simulink model "test_vacc_packetise_jason"  (Simulink 6.2)
settings: Solver=ode45  StartTime=0.0  StopTime=4000  RelTol=1e-3
libraries: xbsIndex_r3 x160, xps_library x10, casper_library x8
settings Model: LastModifiedBy=dsp
settings DebuggingCC: SolverPrmCheckMsg=warning

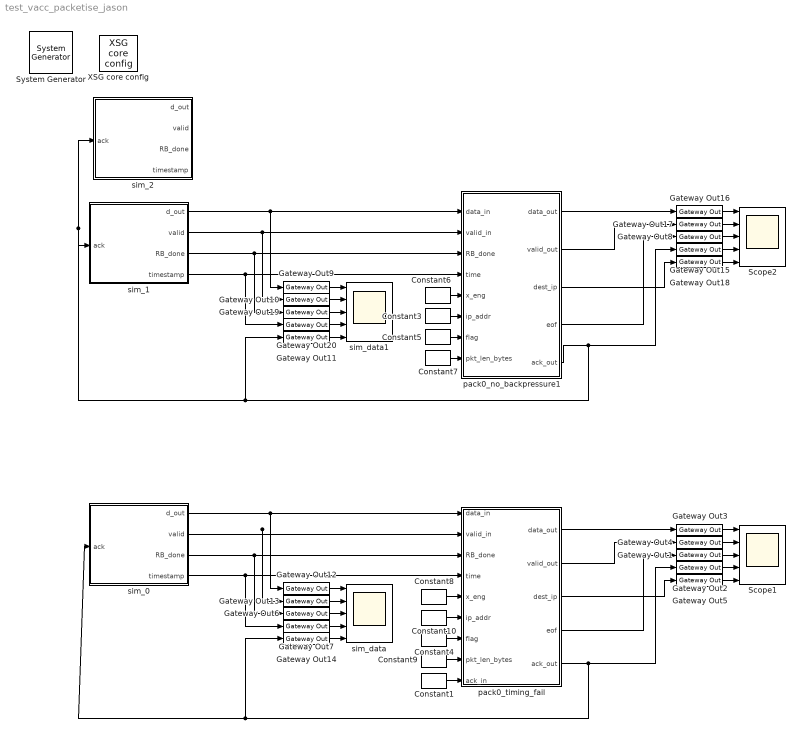
== system test_vacc_packetise_jason ==
  " System Generator" : xbsIndex_r3/ System Generator  Tag=genX  xilinxfamily=Virtex2  part=xc2v1000  speed=-4  package=bg575  synthesis_tool=XST  directory=./netlist  testbench=off  simulink_period=1  sysclk_period=100  incr_netlist=off  trim_vbits=Everywhere in SubSystem  dbl_ovrd=According to Block Masks  core_generation=According to Block Masks  run_coregen=off  deprecated_control=off  eval_field=0
      settings: AttributesFormatString=System\nGenerator
  Constant1 : xbsIndex_r3/Constant  const=1  equ=P=C  arith_type=Boolean  n_bits=32  bin_pt=0  opselect=C  inp2=PCIN>>17  opr=+  inp1=P  carry=CIN  iostate=0  explicit_period=on  period=1  dbl_ovrd=off
  Constant10 : xbsIndex_r3/Constant  const=1  equ=P=C  arith_type=Unsigned  n_bits=32  bin_pt=0  opselect=C  inp2=PCIN>>17  opr=+  inp1=P  carry=CIN  iostate=0  explicit_period=on  period=1  dbl_ovrd=off
  Constant3 : xbsIndex_r3/Constant  const=1  equ=P=C  arith_type=Unsigned  n_bits=32  bin_pt=0  opselect=C  inp2=PCIN>>17  opr=+  inp1=P  carry=CIN  iostate=0  explicit_period=on  period=1  dbl_ovrd=off
  Constant4 : xbsIndex_r3/Constant  const=0  equ=P=C  arith_type=Unsigned  n_bits=32  bin_pt=0  opselect=C  inp2=PCIN>>17  opr=+  inp1=P  carry=CIN  iostate=0  explicit_period=on  period=1  dbl_ovrd=off
  Constant5 : xbsIndex_r3/Constant  const=0  equ=P=C  arith_type=Unsigned  n_bits=32  bin_pt=0  opselect=C  inp2=PCIN>>17  opr=+  inp1=P  carry=CIN  iostate=0  explicit_period=on  period=1  dbl_ovrd=off
  Constant6 : xbsIndex_r3/Constant  const=0  equ=P=C  arith_type=Unsigned  n_bits=32  bin_pt=0  opselect=C  inp2=PCIN>>17  opr=+  inp1=P  carry=CIN  iostate=0  explicit_period=on  period=1  dbl_ovrd=off
  Constant7 : xbsIndex_r3/Constant  const=400  equ=P=C  arith_type=Unsigned  n_bits=32  bin_pt=0  opselect=C  inp2=PCIN>>17  opr=+  inp1=P  carry=CIN  iostate=0  explicit_period=on  period=1  dbl_ovrd=off
  Constant8 : xbsIndex_r3/Constant  const=0  equ=P=C  arith_type=Unsigned  n_bits=16  bin_pt=0  opselect=C  inp2=PCIN>>17  opr=+  inp1=P  carry=CIN  iostate=0  explicit_period=on  period=1  dbl_ovrd=off
  Constant9 : xbsIndex_r3/Constant  const=400  equ=P=C  arith_type=Unsigned  n_bits=32  bin_pt=0  opselect=C  inp2=PCIN>>17  opr=+  inp1=P  carry=CIN  iostate=0  explicit_period=on  period=1  dbl_ovrd=off
  Gateway Out{1..20} (20 alike) : xbsIndex_r3/Gateway Out  output_type=Double  nbits=8  bin_pt=6  arith_type=Boolean  quantization=Truncate  overflow=Wrap  hdl_port=on  timing_constraint=None  locs_specified=off  LOCs={}  needs_fixed_name=off  show_param=off
      settings: xl_area=[0, 0, 0, 0, 0, 0, 0]
  Scope1 : Scope  NumInputPorts=5
      settings: YMin=410.4~-1~-1~-1~0  YMax=453.6~1~1~1~1  SaveName=ScopeData2
  Scope2 : Scope  NumInputPorts=5
      settings: YMin=410.4~-1~-1~-1~0  YMax=453.6~1~1~1~1  SaveName=ScopeData4
  XSG core config : xps_library/XSG core config  Tag=xps:xsg  hw_sys=BEE2_usr  ibob_linux=off  clk_src=sys_clk2x  gpio_clk_io_group=iBOB:sma  gpio_clk_bit_index=0  clk_rate=205  sample_period=1  synthesis_tool=XST  mpc_type=powerpc405
  pack0_no_backpressure1 : Subsystem  mask{vector_len=100}
      mask prompts: vector_len "vector length"
  pack0_timing_fail : Subsystem  mask{vector_len=100}
      mask prompts: vector_len "vector length"
  sim_0 : Subsystem
  sim_1 : Subsystem
  sim_2 : Subsystem
  sim_data : Scope  NumInputPorts=5
      settings: YMin=0~0~0~5~0  YMax=450~1~1~7~1
  sim_data1 : Scope  NumInputPorts=5
      settings: YMin=0~0~0~5~0  YMax=450~1~1~7~1  SaveName=ScopeData5
  wires:
  Gateway Out3/1 -> Scope1/1
  Gateway Out4/1 -> Scope1/2
  Gateway Out1/1 -> Scope1/3
  Gateway Out2/1 -> Scope1/4
  Gateway Out5/1 -> Scope1/5
  sim_0/1(d_out) -> Gateway Out12/1, pack0_timing_fail/1(data_in)
  sim_0/2(valid) -> Gateway Out13/1, pack0_timing_fail/2(valid_in)
  sim_0/3(RB_done) -> Gateway Out6/1, pack0_timing_fail/3(RB_done)
  sim_0/4(timestamp) -> Gateway Out7/1, pack0_timing_fail/4(time)
  Gateway Out12/1 -> sim_data/1
  Gateway Out13/1 -> sim_data/2
  Gateway Out6/1 -> sim_data/3
  Gateway Out7/1 -> sim_data/4
  Gateway Out14/1 -> sim_data/5
  pack0_timing_fail/5(ack_out) -> Gateway Out2/1, Gateway Out14/1, sim_0/1(ack)
  Constant8/1 -> pack0_timing_fail/5(x_eng)
  Constant10/1 -> pack0_timing_fail/6(ip_addr)
  Constant4/1 -> pack0_timing_fail/7(flag)
  pack0_timing_fail/1(data_out) -> Gateway Out3/1
  pack0_timing_fail/2(valid_out) -> Gateway Out4/1
  pack0_timing_fail/4(eof) -> Gateway Out1/1
  pack0_timing_fail/3(dest_ip) -> Gateway Out5/1
  Constant9/1 -> pack0_timing_fail/8(pkt_len_bytes)
  Constant1/1 -> pack0_timing_fail/9(ack_in)
  Gateway Out16/1 -> Scope2/1
  Gateway Out17/1 -> Scope2/2
  Gateway Out8/1 -> Scope2/3
  Gateway Out15/1 -> Scope2/4
  Gateway Out18/1 -> Scope2/5
  sim_1/1(d_out) -> Gateway Out9/1, pack0_no_backpressure1/1(data_in)
  sim_1/2(valid) -> Gateway Out10/1, pack0_no_backpressure1/2(valid_in)
  sim_1/3(RB_done) -> Gateway Out19/1, pack0_no_backpressure1/3(RB_done)
  sim_1/4(timestamp) -> Gateway Out20/1, pack0_no_backpressure1/4(time)
  Gateway Out9/1 -> sim_data1/1
  Gateway Out10/1 -> sim_data1/2
  Gateway Out19/1 -> sim_data1/3
  Gateway Out20/1 -> sim_data1/4
  Gateway Out11/1 -> sim_data1/5
  pack0_no_backpressure1/5(ack_out) -> Gateway Out11/1, sim_1/1(ack), sim_2/1(ack), Gateway Out15/1
  pack0_no_backpressure1/1(data_out) -> Gateway Out16/1
  pack0_no_backpressure1/2(valid_out) -> Gateway Out17/1
  pack0_no_backpressure1/4(eof) -> Gateway Out8/1
  pack0_no_backpressure1/3(dest_ip) -> Gateway Out18/1
  Constant6/1 -> pack0_no_backpressure1/5(x_eng)
  Constant3/1 -> pack0_no_backpressure1/6(ip_addr)
  Constant5/1 -> pack0_no_backpressure1/7(flag)
  Constant7/1 -> pack0_no_backpressure1/8(pkt_len_bytes)

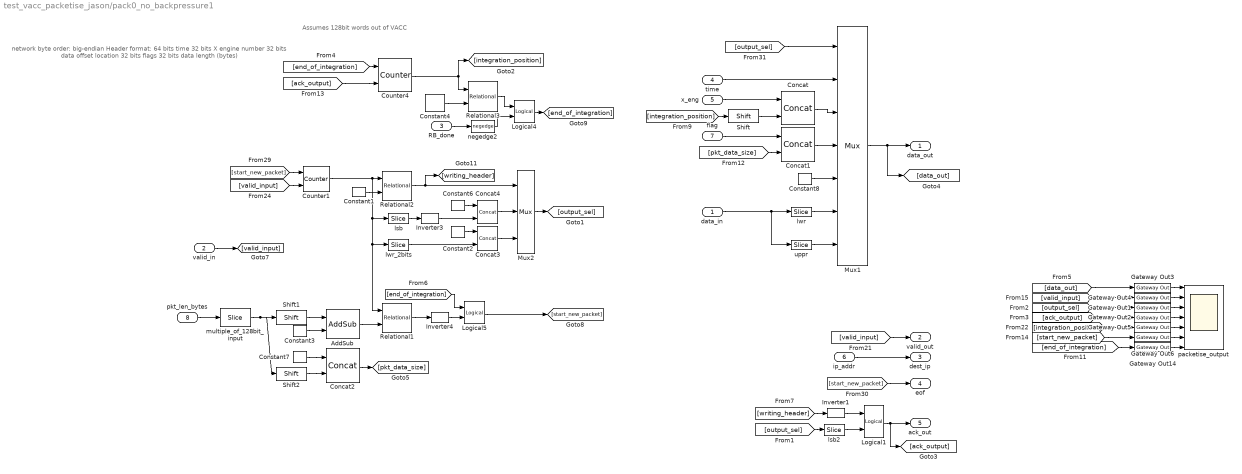
== system test_vacc_packetise_jason/pack0_no_backpressure1 ==
  note: network byte order: big-endian
      |
      | Header format:
      | 64 bits time
      | 32 bits X engine number
      | 32 bits data offset location
      | 32 bits flags
      | 32 bits data length (bytes)
  note: Assumes 128bit words out of VACC
  data_in : Inport  Port=1  LatchInput=off
  valid_in : Inport  Port=2  LatchInput=off
  RB_done : Inport  Port=3  LatchInput=off
  time : Inport  Port=4  LatchInput=off
  x_eng : Inport  Port=5  LatchInput=off
  ip_addr : Inport  Port=6  LatchInput=off
  flag : Inport  Port=7  LatchInput=off
  pkt_len_bytes : Inport  Port=8  LatchInput=off
  AddSub : xbsIndex_r3/AddSub  mode=Addition  precision=Full  arith_type=Unsigned  n_bits=8  bin_pt=2  quantization=Truncate  overflow=Wrap  latency=2  explicit_period=on  period=1  use_carryin=off  use_carryout=off  en=off  dbl_ovrd=off  show_param=off  use_core=on  pipeline=off  use_rpm=on  gen_core=off
      settings: xl_area=[0, 0, 0, 0, 0, 0, 0]
  Concat : xbsIndex_r3/Concat  num_inputs=2  explicit_period=on  period=1  dbl_ovrd=off
  Concat{1..4} (4 alike) : xbsIndex_r3/Concat  num_inputs=2  explicit_period=off  period=1  dbl_ovrd=off
  Constant1 : xbsIndex_r3/Constant  const=2  equ=P=C  arith_type=Unsigned  n_bits=2  bin_pt=0  opselect=C  inp2=PCIN>>17  opr=+  inp1=P  carry=CIN  iostate=0  explicit_period=on  period=1  dbl_ovrd=off
  Constant2 : xbsIndex_r3/Constant  const=0  equ=P=C  arith_type=Unsigned  n_bits=1  bin_pt=0  opselect=C  inp2=PCIN>>17  opr=+  inp1=P  carry=CIN  iostate=0  explicit_period=on  period=1  dbl_ovrd=off
  Constant3 : xbsIndex_r3/Constant  const=2  equ=P=C  arith_type=Unsigned  n_bits=32  bin_pt=0  opselect=C  inp2=PCIN>>17  opr=+  inp1=P  carry=CIN  iostate=0  explicit_period=on  period=1  dbl_ovrd=off
  Constant4 : xbsIndex_r3/Constant  const=2*vector_len-1  equ=P=C  arith_type=Unsigned  n_bits=32  bin_pt=0  opselect=C  inp2=PCIN>>17  opr=+  inp1=P  carry=CIN  iostate=0  explicit_period=off  period=1  dbl_ovrd=off
  Constant6 : xbsIndex_r3/Constant  const=2  equ=P=C  arith_type=Unsigned  n_bits=2  bin_pt=0  opselect=C  inp2=PCIN>>17  opr=+  inp1=P  carry=CIN  iostate=0  explicit_period=on  period=1  dbl_ovrd=off
  Constant7 : xbsIndex_r3/Constant  const=0  equ=P=C  arith_type=Unsigned  n_bits=32-28  bin_pt=0  opselect=C  inp2=PCIN>>17  opr=+  inp1=P  carry=CIN  iostate=0  explicit_period=on  period=1  dbl_ovrd=off
  Constant8 : xbsIndex_r3/Constant  const=0  equ=P=C  arith_type=Unsigned  n_bits=64  bin_pt=0  opselect=C  inp2=PCIN>>17  opr=+  inp1=P  carry=CIN  iostate=0  explicit_period=on  period=1  dbl_ovrd=off
  Counter1 : xbsIndex_r3/Counter  cnt_type=Free Running  n_bits=32  bin_pt=0  arith_type=Unsigned  start_count=0  cnt_to=1023  cnt_by_val=1  operation=Up  explicit_period=on  period=1  load_pin=off  rst=on  en=on  dbl_ovrd=off  show_param=off  use_rpm=on  gen_core=off
      settings: xl_area=[0, 0, 0, 0, 0, 0, 0]
  Counter4 : xbsIndex_r3/Counter  cnt_type=Free Running  n_bits=32  bin_pt=0  arith_type=Unsigned  start_count=0  cnt_to=1023  cnt_by_val=1  operation=Up  explicit_period=on  period=1  load_pin=off  rst=on  en=on  dbl_ovrd=off  show_param=off  use_rpm=on  gen_core=off
      settings: xl_area=[0, 0, 0, 0, 0, 0, 0]
  Gateway Out{1..6,14} (7 alike) : xbsIndex_r3/Gateway Out  output_type=Double  nbits=8  bin_pt=6  arith_type=Boolean  quantization=Truncate  overflow=Wrap  hdl_port=on  timing_constraint=None  locs_specified=off  LOCs={}  needs_fixed_name=off  show_param=off
      settings: xl_area=[0, 0, 0, 0, 0, 0, 0]
  Inverter1 : xbsIndex_r3/Inverter  latency=0  explicit_period=off  period=1  en=off  dbl_ovrd=off  show_param=off
      settings: xl_area=[0, 0, 0, 0, 0, 0, 0]
  Inverter3 : xbsIndex_r3/Inverter  latency=0  explicit_period=off  period=1  en=off  dbl_ovrd=off  show_param=off
      settings: xl_area=[0, 0, 0, 0, 0, 0, 0]
  Inverter4 : xbsIndex_r3/Inverter  latency=0  explicit_period=off  period=1  en=off  dbl_ovrd=off  show_param=off
      settings: xl_area=[0, 0, 0, 0, 0, 0, 0]
  Logical1 : xbsIndex_r3/Logical  logical_function=AND  inputs=2  precision=Full  arith_type=Unsigned  n_bits=8  bin_pt=2  align_bp=on  latency=0  explicit_period=off  period=1  en=off  dbl_ovrd=off  show_param=off
      settings: xl_area=[0, 0, 0, 0, 0, 0, 0]
  Logical4 : xbsIndex_r3/Logical  logical_function=OR  inputs=2  precision=Full  arith_type=Unsigned  n_bits=8  bin_pt=2  align_bp=on  latency=0  explicit_period=off  period=1  en=off  dbl_ovrd=off  show_param=off
      settings: xl_area=[0, 0, 0, 0, 0, 0, 0]
  Logical5 : xbsIndex_r3/Logical  logical_function=OR  inputs=2  precision=Full  arith_type=Unsigned  n_bits=8  bin_pt=2  align_bp=on  latency=0  explicit_period=off  period=1  en=off  dbl_ovrd=off  show_param=off
      settings: xl_area=[0, 0, 0, 0, 0, 0, 0]
  Mux1 : xbsIndex_r3/Mux  inputs=6  precision=Full  arith_type="Signed  (2's comp)"  n_bits=8  bin_pt=2  quantization=Truncate  overflow=Wrap  latency=0  explicit_period=off  period=1  en=off  dbl_ovrd=off  show_param=off  mux_type=off  use_rpm=off  gen_core=off
      settings: xl_area=[0, 0, 0, 0, 0, 0, 0]
  Mux2 : xbsIndex_r3/Mux  inputs=2  precision=Full  arith_type="Signed  (2's comp)"  n_bits=8  bin_pt=2  quantization=Truncate  overflow=Wrap  latency=0  explicit_period=off  period=1  en=off  dbl_ovrd=off  show_param=off  mux_type=off  use_rpm=off  gen_core=off
      settings: xl_area=[0, 0, 0, 0, 0, 0, 0]
  Relational1 : xbsIndex_r3/Relational  mode=a<=b  latency=0  explicit_period=off  period=1  en=off  dbl_ovrd=off  show_param=off
      settings: xl_area=[0, 0, 0, 0, 0, 0, 0]
  Relational2 : xbsIndex_r3/Relational  mode=a<=b  latency=0  explicit_period=off  period=1  en=off  dbl_ovrd=off  show_param=off
      settings: xl_area=[0, 0, 0, 0, 0, 0, 0]
  Relational3 : xbsIndex_r3/Relational  mode=a>=b  latency=0  explicit_period=off  period=1  en=off  dbl_ovrd=off  show_param=off
      settings: xl_area=[0, 0, 0, 0, 0, 0, 0]
  Shift : xbsIndex_r3/Shift  shift_dir=Left  shift_bits=4  precision=Full  arith_type="Signed  (2's comp)"  n_bits=8  bin_pt=2  quantization=Truncate  overflow=Wrap  latency=0  explicit_period=off  period=1  en=off  dbl_ovrd=off  show_param=off
      settings: xl_area=[0, 0, 0, 0, 0, 0, 0]
  Shift1 : xbsIndex_r3/Shift  shift_dir=Left  shift_bits=1  precision=Full  arith_type="Signed  (2's comp)"  n_bits=8  bin_pt=2  quantization=Truncate  overflow=Wrap  latency=2  explicit_period=on  period=1  en=off  dbl_ovrd=off  show_param=off
      settings: xl_area=[0, 0, 0, 0, 0, 0, 0]
  Shift2 : xbsIndex_r3/Shift  shift_dir=Left  shift_bits=4  precision=Full  arith_type="Signed  (2's comp)"  n_bits=8  bin_pt=2  quantization=Truncate  overflow=Wrap  latency=2  explicit_period=on  period=1  en=off  dbl_ovrd=off  show_param=off
      settings: xl_area=[0, 0, 0, 0, 0, 0, 0]
  lsb : xbsIndex_r3/Slice  mode=Lower Bit Location + Width  nbits=1  bit1=0  base1=MSB of Input  bit0=0  base0=LSB of Input  boolean_output=off  explicit_period=off  period=1  dbl_ovrd=off
  lsb2 : xbsIndex_r3/Slice  mode=Lower Bit Location + Width  nbits=1  bit1=0  base1=MSB of Input  bit0=0  base0=LSB of Input  boolean_output=on  explicit_period=off  period=1  dbl_ovrd=off
  lwr : xbsIndex_r3/Slice  mode=Lower Bit Location + Width  nbits=64  bit1=0  base1=MSB of Input  bit0=0  base0=LSB of Input  boolean_output=off  explicit_period=off  period=1  dbl_ovrd=off
  lwr_2bits : xbsIndex_r3/Slice  mode=Lower Bit Location + Width  nbits=2  bit1=0  base1=MSB of Input  bit0=0  base0=LSB of Input  boolean_output=on  explicit_period=off  period=1  dbl_ovrd=off
  multiple_of_128bit_input : xbsIndex_r3/Slice  mode=Two Bit Locations  nbits=64  bit1=31  base1=LSB of Input  bit0=4  base0=LSB of Input  boolean_output=off  explicit_period=off  period=1  dbl_ovrd=off
  negedge2 : casper_library/Misc/negedge  Tag=Rising Edge Detector
  packetise_output : Scope  NumInputPorts=7
      settings: YMin=0~0~0~0~0~0~0  YMax=1200~1~5~1~100~1~1
  uppr : xbsIndex_r3/Slice  mode=Upper Bit Location + Width  nbits=64  bit1=0  base1=MSB of Input  bit0=0  base0=LSB of Input  boolean_output=off  explicit_period=off  period=1  dbl_ovrd=off
  data_out : Outport
  valid_out : Outport  Port=2
  dest_ip : Outport  Port=3
  eof : Outport  Port=4
  ack_out : Outport  Port=5
  wires:
  [ack_output] -> Gateway Out2/1
  AddSub/1 -> Relational1/2
  Shift1/1 -> AddSub/1
  multiple_of_128bit_input/1 -> Shift2/1, Shift1/1
  pkt_len_bytes/1 -> multiple_of_128bit_input/1
  Inverter4/1 -> Logical5/2
  [integration_position] -> Gateway Out5/1
  [end_of_integration] -> Gateway Out14/1
  Gateway Out14/1 -> packetise_output/7
  [valid_input] -> valid_out/1
  [valid_input] -> Gateway Out4/1
  [start_new_packet] -> Gateway Out6/1
  [end_of_integration] -> Logical5/1
  Relational1/1 -> Inverter4/1
  Gateway Out6/1 -> packetise_output/6
  Gateway Out5/1 -> packetise_output/5
  Gateway Out2/1 -> packetise_output/4
  Gateway Out1/1 -> packetise_output/3
  Gateway Out4/1 -> packetise_output/2
  Gateway Out3/1 -> packetise_output/1
  ip_addr/1 -> dest_ip/1
  valid_in/1 -> [valid_input]
  Mux1/1 -> data_out/1, [data_out]
  Logical5/1 -> [start_new_packet]
  Counter1/1 -> Relational2/1, lwr_2bits/1, Relational1/1, lsb/1
  [valid_input] -> Counter1/2
  Constant3/1 -> AddSub/2
  [start_new_packet] -> Counter1/1
  [start_new_packet] -> eof/1
  Relational2/1 -> [writing_header], Mux2/1
  Constant1/1 -> Relational2/2
  Mux2/1 -> [output_sel]
  [output_sel] -> lsb2/1
  Concat2/1 -> [pkt_data_size]
  Shift2/1 -> Concat2/2
  Constant7/1 -> Concat2/1
  [output_sel] -> Mux1/1
  Concat3/1 -> Mux2/3
  lwr_2bits/1 -> Concat3/2
  Constant2/1 -> Concat3/1
  lsb/1 -> Inverter3/1
  Constant6/1 -> Concat4/1
  Concat4/1 -> Mux2/2
  [end_of_integration] -> Counter4/1
  Counter4/1 -> [integration_position], Relational3/1
  [ack_output] -> Counter4/2
  [output_sel] -> Gateway Out1/1
  [data_out] -> Gateway Out3/1
  Logical1/1 -> ack_out/1, [ack_output]
  lsb2/1 -> Logical1/2
  Inverter1/1 -> Logical1/1
  [writing_header] -> Inverter1/1
  Inverter3/1 -> Concat4/2
  Constant4/1 -> Relational3/2
  Logical4/1 -> [end_of_integration]
  Relational3/1 -> Logical4/1
  negedge2/1 -> Logical4/2
  RB_done/1 -> negedge2/1
  data_in/1 -> lwr/1, uppr/1
  lwr/1 -> Mux1/6
  uppr/1 -> Mux1/7
  Constant8/1 -> Mux1/5
  Shift/1 -> Concat/2
  [pkt_data_size] -> Concat1/2
  flag/1 -> Concat1/1
  [integration_position] -> Shift/1
  x_eng/1 -> Concat/1
  Concat1/1 -> Mux1/4
  Concat/1 -> Mux1/3
  time/1 -> Mux1/2

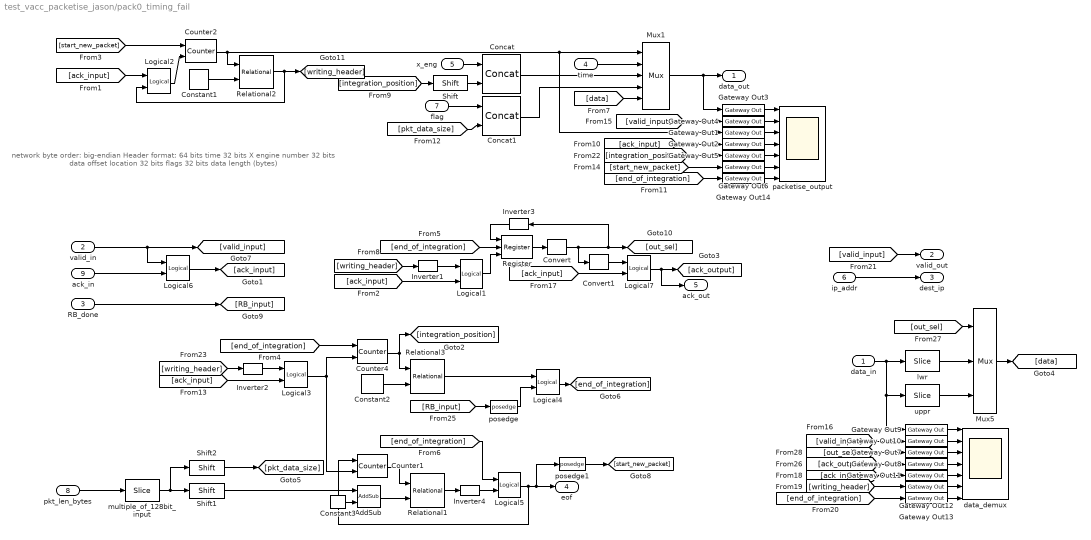
== system test_vacc_packetise_jason/pack0_timing_fail ==
  note: network byte order: big-endian
      |
      | Header format:
      | 64 bits time
      | 32 bits X engine number
      | 32 bits data offset location
      | 32 bits flags
      | 32 bits data length (bytes)
  data_in : Inport  Port=1  LatchInput=off
  valid_in : Inport  Port=2  LatchInput=off
  RB_done : Inport  Port=3  LatchInput=off
  time : Inport  Port=4  LatchInput=off
  x_eng : Inport  Port=5  LatchInput=off
  ip_addr : Inport  Port=6  LatchInput=off
  flag : Inport  Port=7  LatchInput=off
  pkt_len_bytes : Inport  Port=8  LatchInput=off
  ack_in : Inport  Port=9  LatchInput=off
  AddSub : xbsIndex_r3/AddSub  mode=Subtraction  precision=Full  arith_type=Unsigned  n_bits=8  bin_pt=2  quantization=Truncate  overflow=Wrap  latency=2  explicit_period=on  period=1  use_carryin=off  use_carryout=off  en=off  dbl_ovrd=off  show_param=off  use_core=on  pipeline=off  use_rpm=on  gen_core=off
      settings: xl_area=[0, 0, 0, 0, 0, 0, 0]
  Concat : xbsIndex_r3/Concat  num_inputs=2  explicit_period=off  period=1  dbl_ovrd=off
  Concat1 : xbsIndex_r3/Concat  num_inputs=2  explicit_period=off  period=1  dbl_ovrd=off
  Constant1 : xbsIndex_r3/Constant  const=2  equ=P=C  arith_type=Unsigned  n_bits=2  bin_pt=0  opselect=C  inp2=PCIN>>17  opr=+  inp1=P  carry=CIN  iostate=0  explicit_period=off  period=1  dbl_ovrd=off
  Constant2 : xbsIndex_r3/Constant  const=2*vector_len-1  equ=P=C  arith_type=Unsigned  n_bits=32  bin_pt=0  opselect=C  inp2=PCIN>>17  opr=+  inp1=P  carry=CIN  iostate=0  explicit_period=off  period=1  dbl_ovrd=off
  Constant3 : xbsIndex_r3/Constant  const=2  equ=P=C  arith_type=Unsigned  n_bits=32  bin_pt=0  opselect=C  inp2=PCIN>>17  opr=+  inp1=P  carry=CIN  iostate=0  explicit_period=off  period=1  dbl_ovrd=off
  Convert : xbsIndex_r3/Convert  arith_type=Unsigned  n_bits=1  bin_pt=0  quantization=Truncate  overflow=Wrap  latency=0  explicit_period=off  period=1  dbl_ovrd=off  show_param=off  inserted_by_tool=off  pipeline=off
      settings: xl_area=[0, 0, 0, 0, 0, 0, 0]
  Convert1 : xbsIndex_r3/Convert  arith_type=Boolean  n_bits=1  bin_pt=0  quantization=Truncate  overflow=Wrap  latency=0  explicit_period=off  period=1  dbl_ovrd=off  show_param=off  inserted_by_tool=off  pipeline=off
      settings: xl_area=[0, 0, 0, 0, 0, 0, 0]
  Counter1 : xbsIndex_r3/Counter  cnt_type=Free Running  n_bits=32  bin_pt=0  arith_type=Unsigned  start_count=0  cnt_to=1023  cnt_by_val=1  operation=Up  explicit_period=on  period=1  load_pin=off  rst=on  en=on  dbl_ovrd=off  show_param=off  use_rpm=on  gen_core=off
      settings: xl_area=[0, 0, 0, 0, 0, 0, 0]
  Counter2 : xbsIndex_r3/Counter  cnt_type=Free Running  n_bits=2  bin_pt=0  arith_type=Unsigned  start_count=0  cnt_to=1023  cnt_by_val=1  operation=Up  explicit_period=on  period=1  load_pin=off  rst=on  en=on  dbl_ovrd=off  show_param=off  use_rpm=on  gen_core=off
      settings: xl_area=[0, 0, 0, 0, 0, 0, 0]
  Counter4 : xbsIndex_r3/Counter  cnt_type=Free Running  n_bits=32  bin_pt=0  arith_type=Unsigned  start_count=0  cnt_to=1023  cnt_by_val=1  operation=Up  explicit_period=on  period=1  load_pin=off  rst=on  en=on  dbl_ovrd=off  show_param=off  use_rpm=on  gen_core=off
      settings: xl_area=[0, 0, 0, 0, 0, 0, 0]
  Gateway Out{1..14} (14 alike) : xbsIndex_r3/Gateway Out  output_type=Double  nbits=8  bin_pt=6  arith_type=Boolean  quantization=Truncate  overflow=Wrap  hdl_port=on  timing_constraint=None  locs_specified=off  LOCs={}  needs_fixed_name=off  show_param=off
      settings: xl_area=[0, 0, 0, 0, 0, 0, 0]
  Inverter1 : xbsIndex_r3/Inverter  latency=0  explicit_period=off  period=1  en=off  dbl_ovrd=off  show_param=off
      settings: xl_area=[0, 0, 0, 0, 0, 0, 0]
  Inverter2 : xbsIndex_r3/Inverter  latency=0  explicit_period=off  period=1  en=off  dbl_ovrd=off  show_param=off
      settings: xl_area=[0, 0, 0, 0, 0, 0, 0]
  Inverter3 : xbsIndex_r3/Inverter  Orientation=left  latency=0  explicit_period=on  period=1  en=off  dbl_ovrd=off  show_param=off
      settings: xl_area=[0, 0, 0, 0, 0, 0, 0]
  Inverter4 : xbsIndex_r3/Inverter  latency=0  explicit_period=off  period=1  en=off  dbl_ovrd=off  show_param=off
      settings: xl_area=[0, 0, 0, 0, 0, 0, 0]
  Logical{1..3,6..7} (5 alike) : xbsIndex_r3/Logical  logical_function=AND  inputs=2  precision=Full  arith_type=Unsigned  n_bits=8  bin_pt=2  align_bp=on  latency=0  explicit_period=off  period=1  en=off  dbl_ovrd=off  show_param=off
      settings: xl_area=[0, 0, 0, 0, 0, 0, 0]
  Logical4 : xbsIndex_r3/Logical  logical_function=OR  inputs=2  precision=Full  arith_type=Unsigned  n_bits=8  bin_pt=2  align_bp=on  latency=0  explicit_period=off  period=1  en=off  dbl_ovrd=off  show_param=off
      settings: xl_area=[0, 0, 0, 0, 0, 0, 0]
  Logical5 : xbsIndex_r3/Logical  logical_function=OR  inputs=2  precision=Full  arith_type=Unsigned  n_bits=8  bin_pt=2  align_bp=on  latency=0  explicit_period=off  period=1  en=off  dbl_ovrd=off  show_param=off
      settings: xl_area=[0, 0, 0, 0, 0, 0, 0]
  Mux1 : xbsIndex_r3/Mux  inputs=4  precision=Full  arith_type="Signed  (2's comp)"  n_bits=8  bin_pt=2  quantization=Truncate  overflow=Wrap  latency=0  explicit_period=off  period=1  en=off  dbl_ovrd=off  show_param=off  mux_type=off  use_rpm=off  gen_core=off
      settings: xl_area=[0, 0, 0, 0, 0, 0, 0]
  Mux5 : xbsIndex_r3/Mux  inputs=2  precision=Full  arith_type="Signed  (2's comp)"  n_bits=8  bin_pt=2  quantization=Truncate  overflow=Wrap  latency=0  explicit_period=on  period=1  en=off  dbl_ovrd=off  show_param=off  mux_type=off  use_rpm=off  gen_core=off
      settings: xl_area=[0, 0, 0, 0, 0, 0, 0]
  Register : xbsIndex_r3/Register  init=0  reg_only_valid=off  explicit_period=on  period=1  rst=on  en=on  out_en=off  dbl_ovrd=off  show_param=off
      settings: xl_area=[0, 0, 0, 0, 0, 0, 0]
  Relational1 : xbsIndex_r3/Relational  mode=a<=b  latency=0  explicit_period=off  period=1  en=off  dbl_ovrd=off  show_param=off
      settings: xl_area=[0, 0, 0, 0, 0, 0, 0]
  Relational2 : xbsIndex_r3/Relational  mode=a<=b  latency=0  explicit_period=off  period=1  en=off  dbl_ovrd=off  show_param=off
      settings: xl_area=[0, 0, 0, 0, 0, 0, 0]
  Relational3 : xbsIndex_r3/Relational  mode=a>=b  latency=0  explicit_period=off  period=1  en=off  dbl_ovrd=off  show_param=off
      settings: xl_area=[0, 0, 0, 0, 0, 0, 0]
  Shift : xbsIndex_r3/Shift  shift_dir=Left  shift_bits=3  precision=Full  arith_type="Signed  (2's comp)"  n_bits=8  bin_pt=2  quantization=Truncate  overflow=Wrap  latency=0  explicit_period=off  period=1  en=off  dbl_ovrd=off  show_param=off
      settings: xl_area=[0, 0, 0, 0, 0, 0, 0]
  Shift1 : xbsIndex_r3/Shift  shift_dir=Left  shift_bits=1  precision=Full  arith_type="Signed  (2's comp)"  n_bits=8  bin_pt=2  quantization=Truncate  overflow=Wrap  latency=2  explicit_period=on  period=1  en=off  dbl_ovrd=off  show_param=off
      settings: xl_area=[0, 0, 0, 0, 0, 0, 0]
  Shift2 : xbsIndex_r3/Shift  shift_dir=Left  shift_bits=4  precision=Full  arith_type="Signed  (2's comp)"  n_bits=8  bin_pt=2  quantization=Truncate  overflow=Wrap  latency=2  explicit_period=on  period=1  en=off  dbl_ovrd=off  show_param=off
      settings: xl_area=[0, 0, 0, 0, 0, 0, 0]
  data_demux : Scope  NumInputPorts=7
      settings: YMin=410.4~-1~-1~-1~0~-5~-5  YMax=453.6~1~1~1~1~5~5  SaveName=ScopeData3
  lwr : xbsIndex_r3/Slice  mode=Lower Bit Location + Width  nbits=64  bit1=0  base1=MSB of Input  bit0=0  base0=LSB of Input  boolean_output=off  explicit_period=off  period=1  dbl_ovrd=off
  multiple_of_128bit_input : xbsIndex_r3/Slice  mode=Two Bit Locations  nbits=64  bit1=0  base1=MSB of Input  bit0=4  base0=LSB of Input  boolean_output=off  explicit_period=off  period=1  dbl_ovrd=off
  packetise_output : Scope  NumInputPorts=7
      settings: YMin=410.4~-1~-1~-1~0~-5~-5  YMax=453.6~1~1~1~1~5~5
  posedge : casper_library/Misc/posedge  Tag=Rising Edge Detector
  posedge1 : casper_library/Misc/posedge  Tag=Rising Edge Detector
  uppr : xbsIndex_r3/Slice  mode=Upper Bit Location + Width  nbits=64  bit1=0  base1=MSB of Input  bit0=0  base0=LSB of Input  boolean_output=off  explicit_period=off  period=1  dbl_ovrd=off
  data_out : Outport
  valid_out : Outport  Port=2
  dest_ip : Outport  Port=3
  eof : Outport  Port=4
  ack_out : Outport  Port=5
  wires:
  lwr/1 -> Mux5/2
  uppr/1 -> Mux5/3
  [ack_input] -> Logical1/2
  Counter1/1 -> Relational1/1
  Logical5/1 -> Counter1/1, eof/1, posedge1/1
  Constant1/1 -> Relational2/2
  Counter2/1 -> Relational2/1, Mux1/1, Gateway Out1/1
  time/1 -> Mux1/2
  Logical2/1 -> Counter2/2
  Relational2/1 -> Logical2/2, [writing_header]
  [ack_input] -> Logical2/1
  [start_new_packet] -> Counter2/1
  [end_of_integration] -> Counter4/1
  Counter4/1 -> [integration_position], Relational3/1
  Mux1/1 -> data_out/1, Gateway Out3/1
  Mux5/1 -> [data]
  [writing_header] -> Inverter1/1
  Inverter1/1 -> Logical1/1
  x_eng/1 -> Concat/1
  [integration_position] -> Shift/1
  Concat/1 -> Mux1/3
  valid_in/1 -> [valid_input], Logical6/1
  ip_addr/1 -> dest_ip/1
  flag/1 -> Concat1/1
  [pkt_data_size] -> Concat1/2
  Concat1/1 -> Mux1/4
  Logical3/1 -> Counter4/2, Counter1/2
  Gateway Out3/1 -> packetise_output/1
  Gateway Out4/1 -> packetise_output/2
  Gateway Out1/1 -> packetise_output/3
  Gateway Out2/1 -> packetise_output/4
  Gateway Out5/1 -> packetise_output/5
  Gateway Out6/1 -> packetise_output/6
  [data] -> Mux1/5
  Relational1/1 -> Inverter4/1
  [end_of_integration] -> Logical5/1
  Logical6/1 -> [ack_input]
  ack_in/1 -> Logical6/2
  [start_new_packet] -> Gateway Out6/1
  [valid_input] -> Gateway Out4/1
  Gateway Out9/1 -> data_demux/1
  Gateway Out10/1 -> data_demux/2
  Gateway Out7/1 -> data_demux/3
  Gateway Out8/1 -> data_demux/4
  Gateway Out11/1 -> data_demux/5
  Gateway Out12/1 -> data_demux/6
  [valid_input] -> Gateway Out10/1
  Register/1 -> Convert/1
  Inverter3/1 -> Register/1
  [ack_input] -> Logical7/2
  Logical7/1 -> [ack_output], ack_out/1
  Convert1/1 -> Logical7/1
  [ack_input] -> Gateway Out11/1
  [writing_header] -> Gateway Out12/1
  Gateway Out13/1 -> data_demux/7
  [end_of_integration] -> Gateway Out13/1
  data_in/1 -> lwr/1, uppr/1, Gateway Out9/1
  [valid_input] -> valid_out/1
  Convert/1 -> Inverter3/1, [out_sel], Convert1/1
  Constant2/1 -> Relational3/2
  Gateway Out14/1 -> packetise_output/7
  [end_of_integration] -> Gateway Out14/1
  Shift/1 -> Concat/2
  Logical4/1 -> [end_of_integration]
  Relational3/1 -> Logical4/1
  posedge/1 -> Logical4/2
  [integration_position] -> Gateway Out5/1
  Logical1/1 -> Register/3
  [end_of_integration] -> Register/2
  [ack_input] -> Logical3/2
  [writing_header] -> Inverter2/1
  Inverter2/1 -> Logical3/1
  Inverter4/1 -> Logical5/2
  pkt_len_bytes/1 -> multiple_of_128bit_input/1
  multiple_of_128bit_input/1 -> Shift1/1, Shift2/1
  Shift1/1 -> AddSub/1
  AddSub/1 -> Relational1/2
  Constant3/1 -> AddSub/2
  Shift2/1 -> [pkt_data_size]
  posedge1/1 -> [start_new_packet]
  [ack_input] -> Gateway Out2/1
  RB_done/1 -> [RB_input]
  [RB_input] -> posedge/1
  [ack_output] -> Gateway Out8/1
  [out_sel] -> Mux5/1
  [out_sel] -> Gateway Out7/1

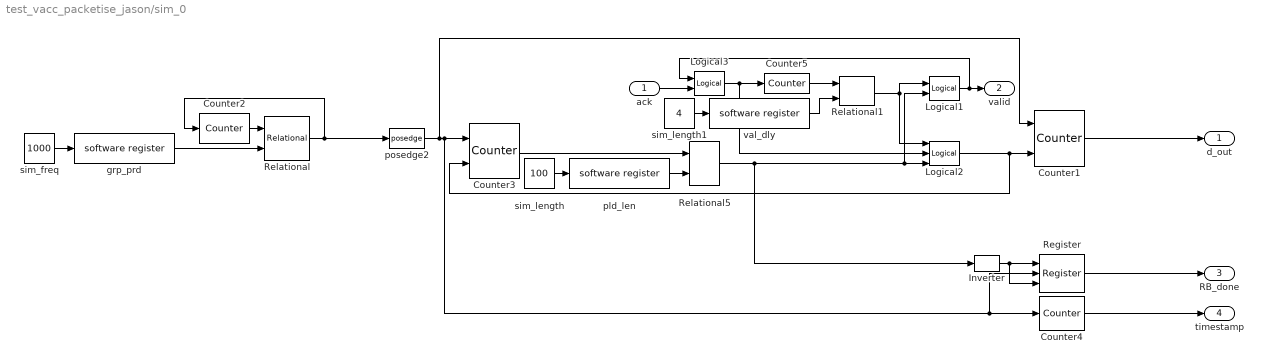
== system test_vacc_packetise_jason/sim_0 ==
  ack : Inport  Port=1  LatchInput=off
  Counter1 : xbsIndex_r3/Counter  cnt_type=Free Running  n_bits=64  bin_pt=0  arith_type=Unsigned  start_count=0  cnt_to=Inf  cnt_by_val=1  operation=Up  explicit_period=off  period=1  load_pin=off  rst=on  en=on  dbl_ovrd=off  show_param=off  use_rpm=off  gen_core=off
      settings: xl_area=[0, 0, 0, 0, 0, 0, 0]
  Counter2 : xbsIndex_r3/Counter  cnt_type=Free Running  n_bits=32  bin_pt=0  arith_type=Unsigned  start_count=1  cnt_to=Inf  cnt_by_val=1  operation=Up  explicit_period=on  period=1  load_pin=off  rst=on  en=off  dbl_ovrd=off  show_param=off  use_rpm=on  gen_core=off
      settings: xl_area=[0, 0, 0, 0, 0, 0, 0]
  Counter3 : xbsIndex_r3/Counter  cnt_type=Free Running  n_bits=32  bin_pt=0  arith_type=Unsigned  start_count=0  cnt_to=1023  cnt_by_val=1  operation=Up  explicit_period=on  period=1  load_pin=off  rst=on  en=on  dbl_ovrd=off  show_param=off  use_rpm=on  gen_core=off
      settings: xl_area=[0, 0, 0, 0, 0, 0, 0]
  Counter4 : xbsIndex_r3/Counter  cnt_type=Free Running  n_bits=64  bin_pt=0  arith_type=Unsigned  start_count=0  cnt_to=1023  cnt_by_val=1  operation=Up  explicit_period=on  period=1  load_pin=off  rst=off  en=on  dbl_ovrd=off  show_param=off  use_rpm=on  gen_core=off
      settings: xl_area=[0, 0, 0, 0, 0, 0, 0]
  Counter5 : xbsIndex_r3/Counter  cnt_type=Free Running  n_bits=32  bin_pt=0  arith_type=Unsigned  start_count=0  cnt_to=1023  cnt_by_val=1  operation=Up  explicit_period=on  period=1  load_pin=off  rst=on  en=off  dbl_ovrd=off  show_param=off  use_rpm=on  gen_core=off
      settings: xl_area=[0, 0, 0, 0, 0, 0, 0]
  Inverter : xbsIndex_r3/Inverter  latency=0  explicit_period=off  period=1  en=off  dbl_ovrd=off  show_param=off
      settings: xl_area=[0, 0, 0, 0, 0, 0, 0]
  Logical1 : xbsIndex_r3/Logical  logical_function=AND  inputs=2  precision=Full  arith_type=Unsigned  n_bits=8  bin_pt=2  align_bp=on  latency=0  explicit_period=off  period=1  en=off  dbl_ovrd=off  show_param=off
      settings: xl_area=[0, 0, 0, 0, 0, 0, 0]
  Logical2 : xbsIndex_r3/Logical  logical_function=AND  inputs=3  precision=Full  arith_type=Unsigned  n_bits=8  bin_pt=2  align_bp=on  latency=0  explicit_period=off  period=1  en=off  dbl_ovrd=off  show_param=off
      settings: xl_area=[0, 0, 0, 0, 0, 0, 0]
  Logical3 : xbsIndex_r3/Logical  logical_function=AND  inputs=2  precision=Full  arith_type=Unsigned  n_bits=8  bin_pt=2  align_bp=on  latency=0  explicit_period=off  period=1  en=off  dbl_ovrd=off  show_param=off
      settings: xl_area=[0, 0, 0, 0, 0, 0, 0]
  Register : xbsIndex_r3/Register  init=0  reg_only_valid=off  explicit_period=off  period=1  rst=on  en=on  out_en=off  dbl_ovrd=off  show_param=off
      settings: xl_area=[0, 0, 0, 0, 0, 0, 0]
  Relational : xbsIndex_r3/Relational  mode=a>=b  latency=0  explicit_period=on  period=1  en=off  dbl_ovrd=off  show_param=off
      settings: xl_area=[0, 0, 0, 0, 0, 0, 0]
  Relational1 : xbsIndex_r3/Relational  mode=a>=b  latency=0  explicit_period=on  period=1  en=off  dbl_ovrd=off  show_param=off
      settings: xl_area=[0, 0, 0, 0, 0, 0, 0]
  Relational5 : xbsIndex_r3/Relational  mode=a<b  latency=0  explicit_period=off  period=1  en=off  dbl_ovrd=off  show_param=off
      settings: xl_area=[0, 0, 0, 0, 0, 0, 0]
  grp_prd : xps_library/software register  Tag=xps:sw_reg  io_dir=From Processor  arith_type=Unsigned  bitwidth=32  bin_pt=0  sample_period=1  gw_name=test_vacc_packetise_jason_sim_0_grp_prd_user_data_out
  pld_len : xps_library/software register  Tag=xps:sw_reg  io_dir=From Processor  arith_type=Unsigned  bitwidth=32  bin_pt=0  sample_period=1  gw_name=test_vacc_packetise_jason_sim_0_pld_len_user_data_out
  posedge2 : casper_library/Misc/pulse_ext/posedge  Tag=Rising Edge Detector
  sim_freq : Constant  Value=1000
  sim_length : Constant  Value=100
  sim_length1 : Constant  Value=4
  val_dly : xps_library/software register  Tag=xps:sw_reg  io_dir=From Processor  arith_type=Unsigned  bitwidth=32  bin_pt=0  sample_period=1  gw_name=test_vacc_packetise_jason_sim_0_val_dly_user_data_out
  d_out : Outport
  valid : Outport  Port=2
  RB_done : Outport  Port=3
  timestamp : Outport  Port=4
  wires:
  Counter2/1 -> Relational/1
  Relational/1 -> Counter2/1, posedge2/1
  Counter1/1 -> d_out/1
  grp_prd/1 -> Relational/2
  sim_freq/1 -> grp_prd/1
  Counter3/1 -> Relational5/1
  posedge2/1 -> Counter1/1, Counter3/1, Counter4/1, Register/2
  sim_length/1 -> pld_len/1
  pld_len/1 -> Relational5/2
  Register/1 -> RB_done/1
  Counter4/1 -> timestamp/1
  Inverter/1 -> Register/1, Register/3
  Relational5/1 -> Inverter/1, Logical2/3, Logical1/2
  Logical2/1 -> Counter1/2, Counter3/2
  Counter5/1 -> Relational1/1
  Logical1/1 -> valid/1, Logical3/1
  sim_length1/1 -> val_dly/1
  val_dly/1 -> Relational1/2
  Relational1/1 -> Logical1/1, Logical2/1
  Logical3/1 -> Counter5/1, Logical2/2
  ack/1 -> Logical3/2

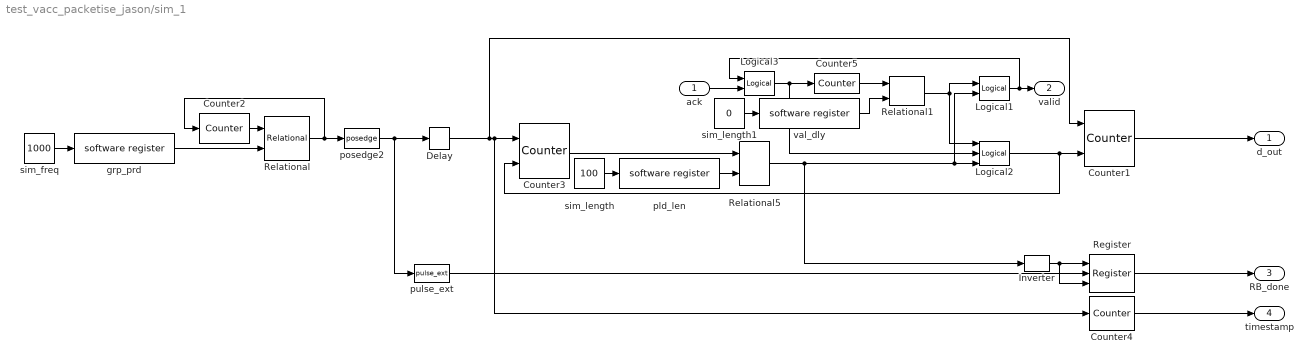
== system test_vacc_packetise_jason/sim_1 ==
  ack : Inport  Port=1  LatchInput=off
  Counter1 : xbsIndex_r3/Counter  cnt_type=Free Running  n_bits=64  bin_pt=0  arith_type=Unsigned  start_count=0  cnt_to=Inf  cnt_by_val=1  operation=Up  explicit_period=off  period=1  load_pin=off  rst=on  en=on  dbl_ovrd=off  show_param=off  use_rpm=off  gen_core=off
      settings: xl_area=[0, 0, 0, 0, 0, 0, 0]
  Counter2 : xbsIndex_r3/Counter  cnt_type=Free Running  n_bits=32  bin_pt=0  arith_type=Unsigned  start_count=1  cnt_to=Inf  cnt_by_val=1  operation=Up  explicit_period=on  period=1  load_pin=off  rst=on  en=off  dbl_ovrd=off  show_param=off  use_rpm=on  gen_core=off
      settings: xl_area=[0, 0, 0, 0, 0, 0, 0]
  Counter3 : xbsIndex_r3/Counter  cnt_type=Free Running  n_bits=32  bin_pt=0  arith_type=Unsigned  start_count=0  cnt_to=1023  cnt_by_val=1  operation=Up  explicit_period=on  period=1  load_pin=off  rst=on  en=on  dbl_ovrd=off  show_param=off  use_rpm=on  gen_core=off
      settings: xl_area=[0, 0, 0, 0, 0, 0, 0]
  Counter4 : xbsIndex_r3/Counter  cnt_type=Free Running  n_bits=64  bin_pt=0  arith_type=Unsigned  start_count=0  cnt_to=1023  cnt_by_val=1  operation=Up  explicit_period=on  period=1  load_pin=off  rst=off  en=on  dbl_ovrd=off  show_param=off  use_rpm=on  gen_core=off
      settings: xl_area=[0, 0, 0, 0, 0, 0, 0]
  Counter5 : xbsIndex_r3/Counter  cnt_type=Free Running  n_bits=32  bin_pt=0  arith_type=Unsigned  start_count=0  cnt_to=1023  cnt_by_val=1  operation=Up  explicit_period=on  period=1  load_pin=off  rst=on  en=off  dbl_ovrd=off  show_param=off  use_rpm=on  gen_core=off
      settings: xl_area=[0, 0, 0, 0, 0, 0, 0]
  Delay : xbsIndex_r3/Delay  latency=4  reg_retiming=on  explicit_period=off  period=1  en=off  accept_only_valid=off  init_zero=on  dbl_ovrd=off  show_param=off
      settings: xl_area=[0, 0, 0, 0, 0, 0, 0]
  Inverter : xbsIndex_r3/Inverter  latency=0  explicit_period=off  period=1  en=off  dbl_ovrd=off  show_param=off
      settings: xl_area=[0, 0, 0, 0, 0, 0, 0]
  Logical1 : xbsIndex_r3/Logical  logical_function=AND  inputs=2  precision=Full  arith_type=Unsigned  n_bits=8  bin_pt=2  align_bp=on  latency=0  explicit_period=off  period=1  en=off  dbl_ovrd=off  show_param=off
      settings: xl_area=[0, 0, 0, 0, 0, 0, 0]
  Logical2 : xbsIndex_r3/Logical  logical_function=AND  inputs=3  precision=Full  arith_type=Unsigned  n_bits=8  bin_pt=2  align_bp=on  latency=0  explicit_period=off  period=1  en=off  dbl_ovrd=off  show_param=off
      settings: xl_area=[0, 0, 0, 0, 0, 0, 0]
  Logical3 : xbsIndex_r3/Logical  logical_function=AND  inputs=2  precision=Full  arith_type=Unsigned  n_bits=8  bin_pt=2  align_bp=on  latency=0  explicit_period=off  period=1  en=off  dbl_ovrd=off  show_param=off
      settings: xl_area=[0, 0, 0, 0, 0, 0, 0]
  Register : xbsIndex_r3/Register  init=0  reg_only_valid=off  explicit_period=off  period=1  rst=on  en=on  out_en=off  dbl_ovrd=off  show_param=off
      settings: xl_area=[0, 0, 0, 0, 0, 0, 0]
  Relational : xbsIndex_r3/Relational  mode=a>=b  latency=0  explicit_period=on  period=1  en=off  dbl_ovrd=off  show_param=off
      settings: xl_area=[0, 0, 0, 0, 0, 0, 0]
  Relational1 : xbsIndex_r3/Relational  mode=a>=b  latency=0  explicit_period=on  period=1  en=off  dbl_ovrd=off  show_param=off
      settings: xl_area=[0, 0, 0, 0, 0, 0, 0]
  Relational5 : xbsIndex_r3/Relational  mode=a<b  latency=0  explicit_period=off  period=1  en=off  dbl_ovrd=off  show_param=off
      settings: xl_area=[0, 0, 0, 0, 0, 0, 0]
  grp_prd : xps_library/software register  Tag=xps:sw_reg  io_dir=From Processor  arith_type=Unsigned  bitwidth=32  bin_pt=0  sample_period=1  gw_name=test_vacc_packetise_jason_sim_1_grp_prd_user_data_out
  pld_len : xps_library/software register  Tag=xps:sw_reg  io_dir=From Processor  arith_type=Unsigned  bitwidth=32  bin_pt=0  sample_period=1  gw_name=test_vacc_packetise_jason_sim_1_pld_len_user_data_out
  posedge2 : casper_library/Misc/pulse_ext/posedge  Tag=Rising Edge Detector
  pulse_ext : casper_library/Misc/pulse_ext  pulse_len=5
  sim_freq : Constant  Value=1000
  sim_length : Constant  Value=100
  sim_length1 : Constant  Value=0
  val_dly : xps_library/software register  Tag=xps:sw_reg  io_dir=From Processor  arith_type=Unsigned  bitwidth=32  bin_pt=0  sample_period=1  gw_name=test_vacc_packetise_jason_sim_1_val_dly_user_data_out
  d_out : Outport
  valid : Outport  Port=2
  RB_done : Outport  Port=3
  timestamp : Outport  Port=4
  wires:
  ack/1 -> Logical3/2
  Logical3/1 -> Logical2/2, Counter5/1
  Relational1/1 -> Logical2/1, Logical1/1
  val_dly/1 -> Relational1/2
  sim_length1/1 -> val_dly/1
  Logical1/1 -> Logical3/1, valid/1
  Counter5/1 -> Relational1/1
  Logical2/1 -> Counter3/2, Counter1/2
  Relational5/1 -> Logical1/2, Logical2/3, Inverter/1
  Inverter/1 -> Register/3, Register/1
  Counter4/1 -> timestamp/1
  pld_len/1 -> Relational5/2
  sim_length/1 -> pld_len/1
  posedge2/1 -> Delay/1, pulse_ext/1
  Counter3/1 -> Relational5/1
  sim_freq/1 -> grp_prd/1
  grp_prd/1 -> Relational/2
  Counter1/1 -> d_out/1
  Relational/1 -> posedge2/1, Counter2/1
  Counter2/1 -> Relational/1
  Register/1 -> RB_done/1
  Delay/1 -> Counter3/1, Counter4/1, Counter1/1
  pulse_ext/1 -> Register/2

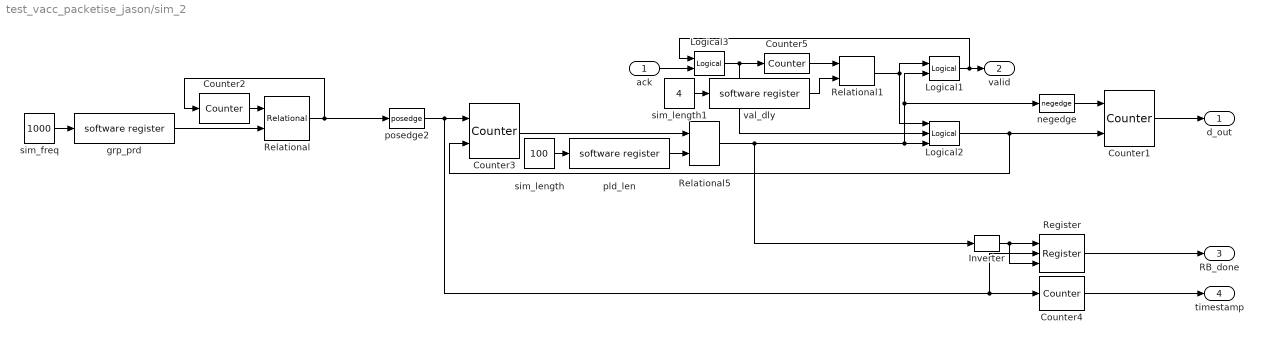
== system test_vacc_packetise_jason/sim_2 ==
  ack : Inport  Port=1  LatchInput=off
  Counter1 : xbsIndex_r3/Counter  cnt_type=Free Running  n_bits=64  bin_pt=0  arith_type=Unsigned  start_count=0  cnt_to=Inf  cnt_by_val=1  operation=Up  explicit_period=off  period=1  load_pin=off  rst=on  en=on  dbl_ovrd=off  show_param=off  use_rpm=off  gen_core=off
      settings: xl_area=[0, 0, 0, 0, 0, 0, 0]
  Counter2 : xbsIndex_r3/Counter  cnt_type=Free Running  n_bits=32  bin_pt=0  arith_type=Unsigned  start_count=1  cnt_to=Inf  cnt_by_val=1  operation=Up  explicit_period=on  period=1  load_pin=off  rst=on  en=off  dbl_ovrd=off  show_param=off  use_rpm=on  gen_core=off
      settings: xl_area=[0, 0, 0, 0, 0, 0, 0]
  Counter3 : xbsIndex_r3/Counter  cnt_type=Free Running  n_bits=32  bin_pt=0  arith_type=Unsigned  start_count=0  cnt_to=1023  cnt_by_val=1  operation=Up  explicit_period=on  period=1  load_pin=off  rst=on  en=on  dbl_ovrd=off  show_param=off  use_rpm=on  gen_core=off
      settings: xl_area=[0, 0, 0, 0, 0, 0, 0]
  Counter4 : xbsIndex_r3/Counter  cnt_type=Free Running  n_bits=64  bin_pt=0  arith_type=Unsigned  start_count=0  cnt_to=1023  cnt_by_val=1  operation=Up  explicit_period=on  period=1  load_pin=off  rst=off  en=on  dbl_ovrd=off  show_param=off  use_rpm=on  gen_core=off
      settings: xl_area=[0, 0, 0, 0, 0, 0, 0]
  Counter5 : xbsIndex_r3/Counter  cnt_type=Free Running  n_bits=32  bin_pt=0  arith_type=Unsigned  start_count=0  cnt_to=1023  cnt_by_val=1  operation=Up  explicit_period=on  period=1  load_pin=off  rst=on  en=off  dbl_ovrd=off  show_param=off  use_rpm=on  gen_core=off
      settings: xl_area=[0, 0, 0, 0, 0, 0, 0]
  Inverter : xbsIndex_r3/Inverter  latency=0  explicit_period=off  period=1  en=off  dbl_ovrd=off  show_param=off
      settings: xl_area=[0, 0, 0, 0, 0, 0, 0]
  Logical1 : xbsIndex_r3/Logical  logical_function=AND  inputs=2  precision=Full  arith_type=Unsigned  n_bits=8  bin_pt=2  align_bp=on  latency=0  explicit_period=off  period=1  en=off  dbl_ovrd=off  show_param=off
      settings: xl_area=[0, 0, 0, 0, 0, 0, 0]
  Logical2 : xbsIndex_r3/Logical  logical_function=AND  inputs=3  precision=Full  arith_type=Unsigned  n_bits=8  bin_pt=2  align_bp=on  latency=0  explicit_period=off  period=1  en=off  dbl_ovrd=off  show_param=off
      settings: xl_area=[0, 0, 0, 0, 0, 0, 0]
  Logical3 : xbsIndex_r3/Logical  logical_function=AND  inputs=2  precision=Full  arith_type=Unsigned  n_bits=8  bin_pt=2  align_bp=on  latency=0  explicit_period=off  period=1  en=off  dbl_ovrd=off  show_param=off
      settings: xl_area=[0, 0, 0, 0, 0, 0, 0]
  Register : xbsIndex_r3/Register  init=0  reg_only_valid=off  explicit_period=off  period=1  rst=on  en=on  out_en=off  dbl_ovrd=off  show_param=off
      settings: xl_area=[0, 0, 0, 0, 0, 0, 0]
  Relational : xbsIndex_r3/Relational  mode=a>=b  latency=0  explicit_period=on  period=1  en=off  dbl_ovrd=off  show_param=off
      settings: xl_area=[0, 0, 0, 0, 0, 0, 0]
  Relational1 : xbsIndex_r3/Relational  mode=a>=b  latency=0  explicit_period=on  period=1  en=off  dbl_ovrd=off  show_param=off
      settings: xl_area=[0, 0, 0, 0, 0, 0, 0]
  Relational5 : xbsIndex_r3/Relational  mode=a<b  latency=0  explicit_period=off  period=1  en=off  dbl_ovrd=off  show_param=off
      settings: xl_area=[0, 0, 0, 0, 0, 0, 0]
  grp_prd : xps_library/software register  Tag=xps:sw_reg  io_dir=From Processor  arith_type=Unsigned  bitwidth=32  bin_pt=0  sample_period=1  gw_name=test_vacc_packetise_jason_sim_2_grp_prd_user_data_out
  negedge : casper_library/Misc/negedge  Tag=Rising Edge Detector
  pld_len : xps_library/software register  Tag=xps:sw_reg  io_dir=From Processor  arith_type=Unsigned  bitwidth=32  bin_pt=0  sample_period=1  gw_name=test_vacc_packetise_jason_sim_2_pld_len_user_data_out
  posedge2 : casper_library/Misc/pulse_ext/posedge  Tag=Rising Edge Detector
  sim_freq : Constant  Value=1000
  sim_length : Constant  Value=100
  sim_length1 : Constant  Value=4
  val_dly : xps_library/software register  Tag=xps:sw_reg  io_dir=From Processor  arith_type=Unsigned  bitwidth=32  bin_pt=0  sample_period=1  gw_name=test_vacc_packetise_jason_sim_2_val_dly_user_data_out
  d_out : Outport
  valid : Outport  Port=2
  RB_done : Outport  Port=3
  timestamp : Outport  Port=4
  wires:
  negedge/1 -> Counter1/1
  Counter2/1 -> Relational/1
  Relational/1 -> Counter2/1, posedge2/1
  Counter1/1 -> d_out/1
  grp_prd/1 -> Relational/2
  sim_freq/1 -> grp_prd/1
  Counter3/1 -> Relational5/1
  posedge2/1 -> Counter3/1, Counter4/1, Register/2
  sim_length/1 -> pld_len/1
  pld_len/1 -> Relational5/2
  Register/1 -> RB_done/1
  Counter4/1 -> timestamp/1
  Inverter/1 -> Register/1, Register/3
  Relational5/1 -> Inverter/1, negedge/1, Logical1/2, Logical2/3
  Logical2/1 -> Counter1/2, Counter3/2
  Counter5/1 -> Relational1/1
  Logical1/1 -> valid/1, Logical3/1
  sim_length1/1 -> val_dly/1
  val_dly/1 -> Relational1/2
  Relational1/1 -> Logical1/1, Logical2/1
  Logical3/1 -> Counter5/1, Logical2/2
  ack/1 -> Logical3/2
